simulink model "robotic_manipulator"  (R2021a)
settings: Solver=VariableStepAuto  StartTime=0.0  StopTime=15  RelTol=1e-2  EnableMultiTasking=on
InitFcn:
  | Ox = 0.2;  %Wspolrzedna x srodka elipsy w m
  | Oy = -0.2;  %Wspolrzedna y srodka elipsy w m
  | 
  | Rx = 0.1;  %promien x ruchu w m
  | Ry = 0.1;  %promien y ruchu w m
  | 
  | To = 8;          %okres obiegu figury w s
  | tx = 0;          %dodatkowy parametr do powtarzania okrazen
  | wd = 2*pi/To;    %pulsacja obiegu w rad/s
  | 
  | zd1 = pi/2;
  | Td1 = 7;
  | wd1 = 2*pi/Td1;
  | 
  | zd2 = pi/3;
  | Td2 = 5;
  | wd2 = 2*pi/Td2;
StopFcn:
  | clear Ox Oy Rx Ry To tx wd zd1 Td1 wd1 zd2 Td2 wd2
libraries: adrc_toolbox_library x2
settings Model: Creator=johnh  LastModifiedBy=PC
settings SolverCC: AlgebraicLoopSolver=TrustRegion
settings DataIOCC: SaveOutput=off  DSMLogging=off  SaveTime=off  ReturnWorkspaceOutputs=off
settings OptimizationCC: LifeSpan=inf
settings DebuggingCC: SFUnexpectedBacktrackingDiag=warning  SFNoUnconditionalDefaultTransitionDiag=warning  SFExecutionAtInitializationDiag=none  SFMachineParentedDataDiag=warning  ArithmeticOperatorsInVariantConditions=warning
settings SFSimCC: SimUseLocalCustomCode=off  CustomCodeUndefinedFunction=UseInterfaceOnly
settings RTWCC: RTWUseLocalCustomCode=off
settings CodeAppCC: StateflowObjectComments=on
settings GRTTargetCC: TargetLangStandard=C89/C90 (ANSI)
settings ConfigComp: CovMetricSettings=dw  CovSaveCumulativeToWorkspaceVar=on  CovSaveSingleToWorkspaceVar=on  CovExternalEMLEnable=off

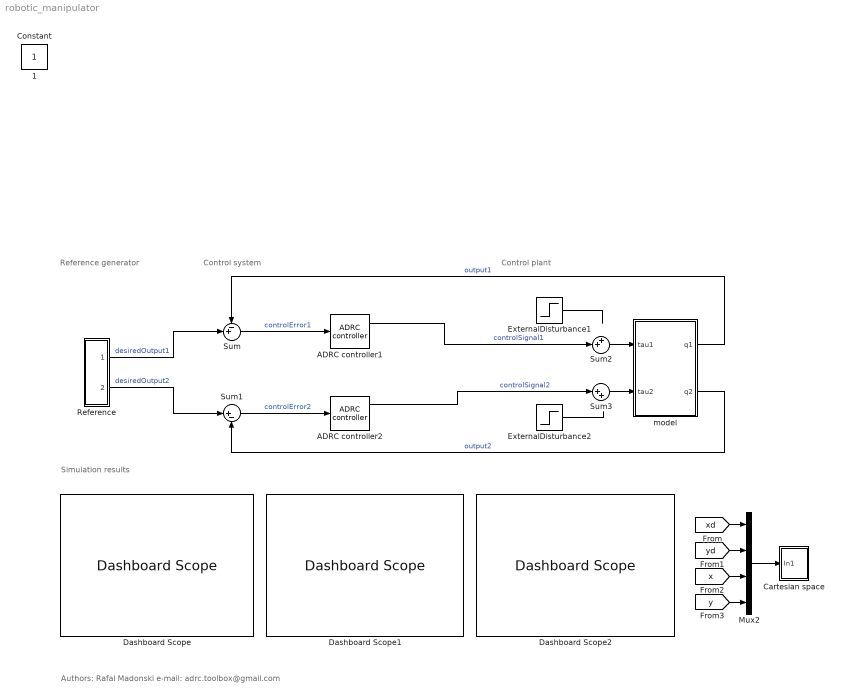
== system robotic_manipulator ==
  note: Authors: Rafal Madonski
      | e-mail: adrc.toolbox@gmail.com
  note: Simulation results
  note: Control system
  note: Control plant
  note: Reference
      | generator
  ADRC controller1 : adrc_toolbox_library/ADRC controller  dynamicsOrder=2  inputGainParameter=8  inputGainSource=Internal  observerBandwidth=100  observerBandwidthSource=Internal  controllerBandwidth=20  controllerBandwidthSource=Internal  saturationEnabled=on  UpperLimit=10  LowerLimit=-10  deadTimeEnabled=off  deadTime=0.3  observerOutputEnabled=on  observerOutputChoice=Estimated control error
      settings: SourceProductName=ADRC toolbox
  ADRC controller2 : adrc_toolbox_library/ADRC controller  dynamicsOrder=2  inputGainParameter=8  inputGainSource=Internal  observerBandwidth=100  observerBandwidthSource=Internal  controllerBandwidth=20  controllerBandwidthSource=Internal  saturationEnabled=on  UpperLimit=10  LowerLimit=-10  deadTimeEnabled=off  deadTime=2  observerOutputEnabled=on  observerOutputChoice=Estimated control error
      settings: SourceProductName=ADRC toolbox
  Cartesian space : Subsystem  mask(Mutiple XY Graph){number_of_trajectories=2, axis_limits=[0 0.4 -0.45 -0.05], sample_time=0.1}
      mask prompts: number_of_trajectories "Number of Trajectories"; axis_limits "Axis Limits"; sample_time "Sample Time"
      mask Display: plot([.05 .95 .95 .05 .05],[.45 .45 .95 .95 .45], 0.5+cos(0:0.1:2*pi)*0.3,0.7+sin(0:0.1:2*pi)*0.2)
  Dashboard Scope : DashboardScope  Ymin=0  Ymax=100
  Dashboard Scope1 : DashboardScope  Ymin=0  Ymax=100
  Dashboard Scope2 : DashboardScope  Ymin=-50  Ymax=50
  ExternalDisturbance1 : Step  Time=90  After=-1.4e-4  SampleTime=0
  ExternalDisturbance2 : Step  Time=130  After=-0.7e-4  SampleTime=0
  Mux2 : Mux
  Reference : Subsystem
  Sum : Sum  Inputs=-+|
  Sum1 : Sum  Inputs=|+-
  Sum2 : Sum  Inputs=++|
  Sum3 : Sum  Inputs=|++
  model : Subsystem
  1 : Constant  IOType=siggen
  Constant : Constant  IOType=siggen
  wires:
  model/1(q1) -> Sum/1  "output1"
  Reference/1(qd1) -> Sum/2  "desiredOutput1"
  Sum/1 -> ADRC controller1/1  "controlError1"
  ADRC controller2/1 -> Sum3/1  "controlSignal2"
  Reference/2(qd2) -> Sum1/1  "desiredOutput2"
  model/2(q2) -> Sum1/2  "output2"
  ADRC controller1/1 -> Sum2/2  "controlSignal1"
  ExternalDisturbance1/1 -> ?
  ExternalDisturbance2/1 -> ?
  Sum2/1 -> model/1(tau1)
  Sum3/1 -> model/2(tau2)
  Sum1/1 -> ADRC controller2/1  "controlError2"
  Mux2/1 -> Cartesian space/1(In1)
  [xd] -> Mux2/1
  [yd] -> Mux2/2
  [x] -> Mux2/3
  [y] -> Mux2/4

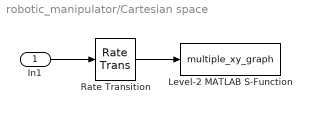
== system robotic_manipulator/Cartesian space ==
  In1 : Inport
  Level-2 MATLAB S-Function : M-S-Function  FunctionName=multiple_xy_graph  Parameters=number_of_trajectories,axis_limits
  Rate Transition : RateTransition  OutPortSampleTime=sample_time
  wires:
  In1/1 -> Rate Transition/1
  Rate Transition/1 -> Level-2 MATLAB S-Function/1

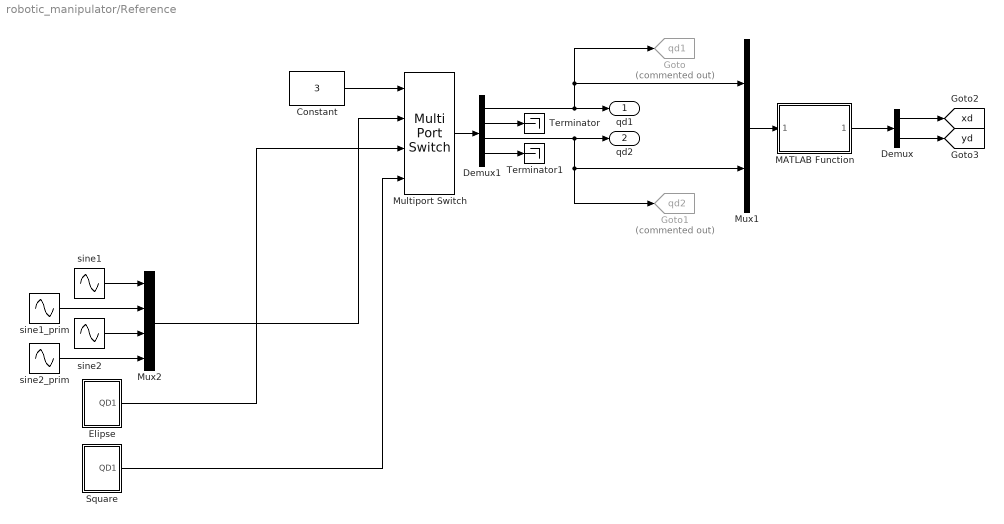
== system robotic_manipulator/Reference ==
  Constant : Constant  Value=3
  Demux : Demux  Outputs=2
  Demux1 : Demux
  Elipse : Subsystem
  Goto : Goto  Commented=on  GotoTag=qd1  TagVisibility=global
  Goto1 : Goto  Commented=on  GotoTag=qd2  TagVisibility=global
  MATLAB Function : MATLAB Function  TreatAsAtomicUnit=on
  Multiport Switch : MultiPortSwitch
  Mux1 : Mux  Inputs=2
  Mux2 : Mux
  Square : Subsystem
  Terminator : Terminator
  Terminator1 : Terminator
  sine1 : Sin  Amplitude=zd1  Frequency=wd1  SampleTime=0
  sine1_prim : Sin  Amplitude=zd1*wd1  Frequency=wd1  Phase=pi/2  SampleTime=0
  sine2 : Sin  Amplitude=zd2  Frequency=wd2  SampleTime=0
  sine2_prim : Sin  Amplitude=zd2*wd2  Frequency=wd2  Phase=pi/2  SampleTime=0
  qd1 : Outport  VectorParamsAs1DForOutWhenUnconnected=off
  qd2 : Outport  Port=2  VectorParamsAs1DForOutWhenUnconnected=off
  tag scope: xd=global, yd=global
  wires:
  Constant/1 -> Multiport Switch/1
  sine1/1 -> Mux2/1
  sine1_prim/1 -> Mux2/2
  sine2/1 -> Mux2/3
  sine2_prim/1 -> Mux2/4
  Multiport Switch/1 -> Demux1/1
  Demux1/1 -> Goto/1, Mux1/1, qd1/1
  Demux1/3 -> Goto1/1, Mux1/2, qd2/1
  Demux1/2 -> Terminator/1
  Demux1/4 -> Terminator1/1
  Mux1/1 -> MATLAB Function/1(wejscie)
  MATLAB Function/1(wyjscie) -> Demux/1
  Demux/1 -> [xd]
  Demux/2 -> [yd]
  Mux2/1 -> Multiport Switch/2
  Square/1(QD1) -> Multiport Switch/4
  Elipse/1(QD1) -> Multiport Switch/3

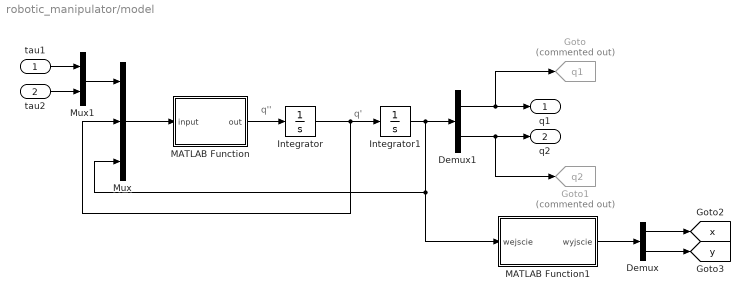
== system robotic_manipulator/model ==
  note: q''
  note: q'
  tau1 : Inport
  tau2 : Inport  Port=2
  Demux : Demux  Outputs=2
  Demux1 : Demux  Outputs=2
  Goto : Goto  Commented=on  GotoTag=q1  TagVisibility=global
  Goto1 : Goto  Commented=on  GotoTag=q2  TagVisibility=global
  Integrator : Integrator  InitialCondition=[0;0]
  Integrator1 : Integrator  InitialCondition=[0;0]
  MATLAB Function : MATLAB Function  TreatAsAtomicUnit=on
  MATLAB Function1 : MATLAB Function  TreatAsAtomicUnit=on
  Mux : Mux  Inputs=3
  Mux1 : Mux  Inputs=2
  q1 : Outport  VectorParamsAs1DForOutWhenUnconnected=off
  q2 : Outport  Port=2  VectorParamsAs1DForOutWhenUnconnected=off
  tag scope: x=global, y=global
  wires:
  MATLAB Function/1(out) -> Integrator/1
  Integrator/1 -> Integrator1/1, Mux/2
  Integrator1/1 -> Demux1/1, MATLAB Function1/1(wejscie), Mux/3
  Demux1/1 -> Goto/1, q1/1
  Mux/1 -> MATLAB Function/1(input)
  Demux1/2 -> Goto1/1, q2/1
  tau2/1 -> Mux1/2
  tau1/1 -> Mux1/1
  Mux1/1 -> Mux/1
  MATLAB Function1/1(wyjscie) -> Demux/1
  Demux/1 -> [x]
  Demux/2 -> [y]

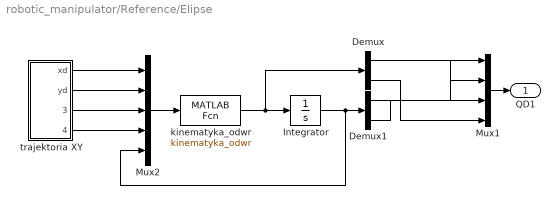
== system robotic_manipulator/Reference/Elipse ==
  Demux : Demux  Outputs=2
  Demux1 : Demux  Outputs=2
  Integrator : Integrator
  Mux1 : Mux
  Mux2 : Mux  Inputs=5
  kinematyka_odwr : MATLABFcn  MATLABFcn=kinematyka_odwr  OutputDimensions=2
  trajektoria XY : Subsystem
  QD1 : Outport  VectorParamsAs1DForOutWhenUnconnected=off
  wires:
  Mux2/1 -> kinematyka_odwr/1
  kinematyka_odwr/1 -> Integrator/1, Demux/1
  trajektoria XY/1(xd) -> Mux2/1
  trajektoria XY/2(yd) -> Mux2/2
  Integrator/1 -> Mux2/5, Demux1/1
  Mux1/1 -> QD1/1
  Demux/1 -> Mux1/2
  Demux/2 -> Mux1/4
  Demux1/1 -> Mux1/1
  Demux1/2 -> Mux1/3
  trajektoria XY/3(xd_prim) -> Mux2/3
  trajektoria XY/4(yd_prim) -> Mux2/4

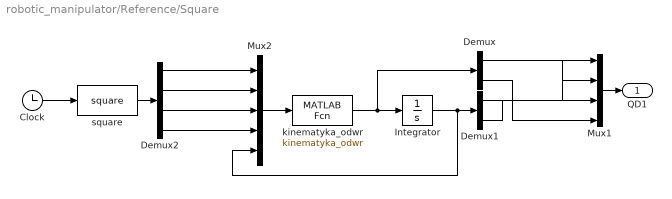
== system robotic_manipulator/Reference/Square ==
  Clock : Clock
  Demux : Demux  Outputs=2
  Demux1 : Demux  Outputs=2
  Demux2 : Demux
  Integrator : Integrator
  Mux1 : Mux
  Mux2 : Mux  Inputs=5
  kinematyka_odwr : MATLABFcn  MATLABFcn=kinematyka_odwr  OutputDimensions=2
  square : MATLABFcn  MATLABFcn=square  OutputDimensions=4
  QD1 : Outport  VectorParamsAs1DForOutWhenUnconnected=off
  wires:
  Demux1/2 -> Mux1/3
  Demux1/1 -> Mux1/1
  Demux/2 -> Mux1/4
  Demux/1 -> Mux1/2
  Mux1/1 -> QD1/1
  Integrator/1 -> Demux1/1, Mux2/5
  kinematyka_odwr/1 -> Demux/1, Integrator/1
  Mux2/1 -> kinematyka_odwr/1
  Clock/1 -> square/1
  square/1 -> Demux2/1
  Demux2/1 -> Mux2/1
  Demux2/2 -> Mux2/2
  Demux2/3 -> Mux2/3
  Demux2/4 -> Mux2/4

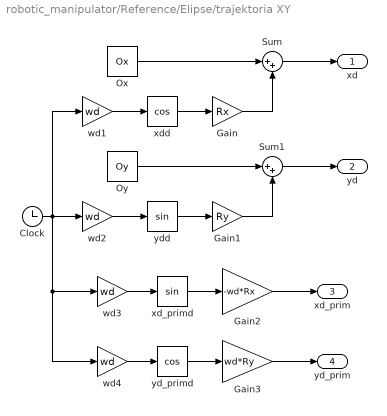
== system robotic_manipulator/Reference/Elipse/trajektoria XY ==
  Clock : Clock
  Gain : Gain  Gain=Rx
  Gain1 : Gain  Gain=Ry
  Gain2 : Gain  Gain=-wd*Rx
  Gain3 : Gain  Gain=wd*Ry
  Ox : Constant  Value=Ox
  Oy : Constant  Value=Oy
  Sum : Sum  Inputs=|++
  Sum1 : Sum  Inputs=|++
  wd{1..4} (4 alike) : Gain  Gain=wd
  xd_primd : Trigonometry
  xdd : Trigonometry  Operator=cos
  yd_primd : Trigonometry  Operator=cos
  ydd : Trigonometry
  xd : Outport  VectorParamsAs1DForOutWhenUnconnected=off
  yd : Outport  Port=2  VectorParamsAs1DForOutWhenUnconnected=off
  xd_prim : Outport  Port=3  VectorParamsAs1DForOutWhenUnconnected=off
  yd_prim : Outport  Port=4  VectorParamsAs1DForOutWhenUnconnected=off
  wires:
  Ox/1 -> Sum/1
  Oy/1 -> Sum1/1
  xdd/1 -> Gain/1
  Gain/1 -> Sum/2
  ydd/1 -> Gain1/1
  Gain1/1 -> Sum1/2
  wd1/1 -> xdd/1
  wd2/1 -> ydd/1
  Clock/1 -> wd2/1, wd1/1, wd3/1, wd4/1
  Sum/1 -> xd/1
  Sum1/1 -> yd/1
  wd4/1 -> yd_primd/1
  wd3/1 -> xd_primd/1
  xd_primd/1 -> Gain2/1
  yd_primd/1 -> Gain3/1
  Gain2/1 -> xd_prim/1
  Gain3/1 -> yd_prim/1

== matlab function robotic_manipulator/model/MATLAB Function ==
  data: input input; out output
function out = pmxr(input)

m1 = 0.7;
m2 = 0.5;
I1 = 0.083;
I2 = 0.04;
L1 = 0.25;
L2 = 0.18;
b1 = 0.1;
b2 = 0.1;
g = 9.81;
fc = 0.1;

tau1 = input(1); 
tau2 = input(2);

qprim1 = input(3);
qprim2 = input(4);

q1 = input(5);
q2 = input(6);

tau = [tau1 ; tau2]; 
qprim = [qprim1 ; qprim2];

M11 = m1*L1*L1 + I1 + m2*L2*L2 + I2 + 4*m2*L1*L1 + 4*m2*L1*L2*cos(q2);
M12 = m2*L2*L2 + I2 + 2*m2*L1*L2*cos(q2);
M21 = m2*L2*L2 + I2 + 2*m2*L1*L2*cos(q2);
M22 = m2*L2*L2 + I2;

M = [M11 M12 ; M21 M22]; %macierz mas

C11 = -2*m2*L1*L2*qprim2*sin(q2);
C12 = -2*m2*L1*L2*(qprim1+qprim2)*sin(q2);
C21 = 2*m2*L1*L2*qprim1*sin(q2);
C22 = 0;

C = [C11 C12 ; C21 C22]; %macierz sil coriolisa i odsrodkowych

G1 = (m1*L1 + 2*m2*L1)*g*cos(q1) + m2*L2*g*cos(q1 + q2);
G2 = m2*L2*g*cos(q1 + q2);

G = [G1 ; G2]; %wektor grawitacji

F1 = fc*sign(qprim1) + b1*qprim1;
F2 = fc*sign(qprim2) + b2*qprim2;

F = [F1 ; F2]; %wektor tarcia

%iM = inv(M);

qbis = M\tau - M\(C*qprim) - M\F - M\G;

out = qbis;

== matlab function robotic_manipulator/model/MATLAB Function1 ==
  data: wejscie input; wyjscie output
function wyjscie = kinematyka(wejscie)

L1 = 0.25;
L2 = 0.18;

q1 = wejscie(1);
q2 = wejscie(2);

wyjscie = [L1*sin(q1)+L2*sin(q1+q2) ; -L1*cos(q1)-L2*cos(q1+q2)];

== matlab function robotic_manipulator/Reference/MATLAB Function ==
  data: wejscie input; wyjscie output
function wyjscie = kinematyka(wejscie)

L1 = 0.25;
L2 = 0.18;

q1 = wejscie(1);
q2 = wejscie(2);

wyjscie = [L1*sin(q1)+L2*sin(q1+q2) ; -L1*cos(q1)-L2*cos(q1+q2)];
